simulink library "AEMS_Standard_Library"  (R2016b)
settings: Solver=ode45  StartTime=0.0  StopTime=10.0  RelTol=1e-3
undefined symbols (not defined in the file or in its folder): BkPY, carto, Cbx_extegr, Cbx_lpegrsys, Cbx_portegr, Cnx_bnk_nr_conf, Cnx_cyl_nr_conf, ConfigManagement, configuration_management, Cxx_dcm_io_tmr_end_xxxx, Cxx_dcm_rt_tmr_end, Cxx_DID_xxxx_IO_max, Cxx_DID_xxxx_IO_min, Cxx_egrhsofs, Cxx_vmaniegi, DEM_DEBOUNCE_FREEZE, DEM_DTR_CTL_INVISIBLE, DEM_DTR_CTL_NORMAL, Dem_DtrId2_XXX, Dem_DtrId3_XXX, Dem_DtrId4_XXX, Dem_DtrId5_XXX, Dem_DtrId6_XXX, Dem_DtrId7_XXX, Dem_DtrId8_XXX, Dem_DtrId9_XXX, Dem_DtrId_XXX, Dem_EnableConditionId2_XXX, Dem_EnableConditionId3_XXX, Dem_EnableConditionId4_XXX, Dem_EnableConditionId5_XXX, Dem_EnableConditionId6_XXX, Dem_EnableConditionId7_XXX, Dem_EnableConditionId8_XXX, Dem_EnableConditionId_XXX, Dem_EventId, Dem_EventId2_XXX, Dem_EventId3_XXX, Dem_EventId4_XXX, Dem_EventId5_XXX, Dem_EventId6_XXX, Dem_EventId7_XXX, Dem_EventId8_XXX, Dem_EventId9_XXX, Dem_EventId_Device_Faulttype, Dem_EventId_XXX, DEM_IUMPR_GENERAL_DENOMINATOR, DEM_OPCYC_IGNITION, Dem_RatioId2_XXX, Dem_RatioId3_XXX, Dem_RatioId4_XXX, Dem_RatioId5_XXX, Dem_RatioId6_XXX, Dem_RatioId7_XXX, Dem_RatioId8_XXX, Dem_RatioId_XXX, Dem_StorageConditionId2_XXX, Dem_StorageConditionId3_XXX, Dem_StorageConditionId4_XXX, Dem_StorageConditionId5_XXX ... (+65)
libraries: AEMS_Standard_Library x477, simulink x2
(part 21 of 39)

== system AEMS_Standard_Library/SUB/AEMS_DEM_COUNTER_BASED_DEBOUNCE_6D ==
  note: DemDebounceBehavior
  flag_set : Inport
  conditionfulfilled : Inport  Port=2
  prefailed : Inport  Port=3
  prepassed : Inport  Port=4
  reseteventdebounce : Inport  Port=5
  AEMS_DEM_COUNTER_BASED_DEBOUNCE_CALL1 : Subsystem
  AEMS_DEM_COUNTER_BASED_DEBOUNCE_CALL2 : Subsystem
  AEMS_DEM_COUNTER_BASED_DEBOUNCE_CALL3 : Subsystem
  AEMS_DEM_COUNTER_BASED_DEBOUNCE_CALL4 : Subsystem
  AEMS_DEM_COUNTER_BASED_DEBOUNCE_CALL5 : Subsystem
  AEMS_DEM_COUNTER_BASED_DEBOUNCE_CALL6 : Subsystem
  DemCounterDecrementStepSize : Constant  Value=DemCounterDecrementStepSize
  DemCounterFailedThreshold : Constant  Value=DemCounterFailedThreshold
  DemCounterIncrementStepSize : Constant  Value=DemCounterIncrementStepSize
  DemCounterJumpDown : Constant  Value=DemCounterJumpDown
  DemCounterJumpDownValue : Constant  Value=DemCounterJumpDownValue
  DemCounterJumpUp : Constant  Value=DemCounterJumpUp
  DemCounterJumpUpValue : Constant  Value=DemCounterJumpUpValue
  DemCounterPassedThreshold : Constant  Value=DemCounterPassedThreshold
  DemDebounceBehavior : Constant  Value=[0,0,0,0,0,0]  OutDataTypeStr=uint8
  Demux{,1..13} (14 alike) : Demux  Outputs=6
  Mux : Mux  Inputs=6
  Mux1 : Mux  Inputs=6
  Mux2 : Mux  Inputs=6
  debouncevalue : Outport
  failed : Outport  Port=2
  passed : Outport  Port=3
  wires:
  AEMS_DEM_COUNTER_BASED_DEBOUNCE_CALL6/3(passed) -> Mux/6
  AEMS_DEM_COUNTER_BASED_DEBOUNCE_CALL5/3(passed) -> Mux/5
  AEMS_DEM_COUNTER_BASED_DEBOUNCE_CALL6/2(failed) -> Mux2/6
  AEMS_DEM_COUNTER_BASED_DEBOUNCE_CALL5/2(failed) -> Mux2/5
  AEMS_DEM_COUNTER_BASED_DEBOUNCE_CALL6/1(debouncevalue) -> Mux1/6
  AEMS_DEM_COUNTER_BASED_DEBOUNCE_CALL5/1(debouncevalue) -> Mux1/5
  Demux7/6 -> AEMS_DEM_COUNTER_BASED_DEBOUNCE_CALL6/13(DemCounterJumpDownValue)
  Demux7/5 -> AEMS_DEM_COUNTER_BASED_DEBOUNCE_CALL5/13(DemCounterJumpDownValue)
  Demux6/6 -> AEMS_DEM_COUNTER_BASED_DEBOUNCE_CALL6/12(DemCounterJumpDown)
  Demux6/5 -> AEMS_DEM_COUNTER_BASED_DEBOUNCE_CALL5/12(DemCounterJumpDown)
  Demux5/6 -> AEMS_DEM_COUNTER_BASED_DEBOUNCE_CALL6/11(DemCounterDecrementStepSize)
  Demux5/5 -> AEMS_DEM_COUNTER_BASED_DEBOUNCE_CALL5/11(DemCounterDecrementStepSize)
  Demux10/6 -> AEMS_DEM_COUNTER_BASED_DEBOUNCE_CALL6/10(DemCounterPassedThreshold)
  Demux10/5 -> AEMS_DEM_COUNTER_BASED_DEBOUNCE_CALL5/10(DemCounterPassedThreshold)
  Demux9/6 -> AEMS_DEM_COUNTER_BASED_DEBOUNCE_CALL6/9(DemCounterJumpUpValue)
  Demux9/5 -> AEMS_DEM_COUNTER_BASED_DEBOUNCE_CALL5/9(DemCounterJumpUpValue)
  Demux8/6 -> AEMS_DEM_COUNTER_BASED_DEBOUNCE_CALL6/8(DemCounterJumpUp)
  Demux8/5 -> AEMS_DEM_COUNTER_BASED_DEBOUNCE_CALL5/8(DemCounterJumpUp)
  Demux13/6 -> AEMS_DEM_COUNTER_BASED_DEBOUNCE_CALL6/7(DemCounterIncrementStepSize)
  Demux13/5 -> AEMS_DEM_COUNTER_BASED_DEBOUNCE_CALL5/7(DemCounterIncrementStepSize)
  Demux12/6 -> AEMS_DEM_COUNTER_BASED_DEBOUNCE_CALL6/6(DemCounterFailedThreshold)
  Demux12/5 -> AEMS_DEM_COUNTER_BASED_DEBOUNCE_CALL5/6(DemCounterFailedThreshold)
  Demux11/6 -> AEMS_DEM_COUNTER_BASED_DEBOUNCE_CALL6/5(DemDebounceBehavior)
  Demux11/5 -> AEMS_DEM_COUNTER_BASED_DEBOUNCE_CALL5/5(DemDebounceBehavior)
  Demux4/6 -> AEMS_DEM_COUNTER_BASED_DEBOUNCE_CALL6/4(reseteventdebounce)
  Demux4/5 -> AEMS_DEM_COUNTER_BASED_DEBOUNCE_CALL5/4(reseteventdebounce)
  Demux3/6 -> AEMS_DEM_COUNTER_BASED_DEBOUNCE_CALL6/3(prepassed)
  Demux3/5 -> AEMS_DEM_COUNTER_BASED_DEBOUNCE_CALL5/3(prepassed)
  Demux2/6 -> AEMS_DEM_COUNTER_BASED_DEBOUNCE_CALL6/2(prefailed)
  Demux2/5 -> AEMS_DEM_COUNTER_BASED_DEBOUNCE_CALL5/2(prefailed)
  Demux1/6 -> AEMS_DEM_COUNTER_BASED_DEBOUNCE_CALL6/1(conditionfulfilled)
  Demux1/5 -> AEMS_DEM_COUNTER_BASED_DEBOUNCE_CALL5/1(conditionfulfilled)
  Demux/6 -> AEMS_DEM_COUNTER_BASED_DEBOUNCE_CALL6/Enable
  Demux/5 -> AEMS_DEM_COUNTER_BASED_DEBOUNCE_CALL5/Enable
  AEMS_DEM_COUNTER_BASED_DEBOUNCE_CALL4/3(passed) -> Mux/4
  AEMS_DEM_COUNTER_BASED_DEBOUNCE_CALL4/2(failed) -> Mux2/4
  AEMS_DEM_COUNTER_BASED_DEBOUNCE_CALL4/1(debouncevalue) -> Mux1/4
  Demux7/4 -> AEMS_DEM_COUNTER_BASED_DEBOUNCE_CALL4/13(DemCounterJumpDownValue)
  Demux6/4 -> AEMS_DEM_COUNTER_BASED_DEBOUNCE_CALL4/12(DemCounterJumpDown)
  Demux5/4 -> AEMS_DEM_COUNTER_BASED_DEBOUNCE_CALL4/11(DemCounterDecrementStepSize)
  Demux10/4 -> AEMS_DEM_COUNTER_BASED_DEBOUNCE_CALL4/10(DemCounterPassedThreshold)
  Demux9/4 -> AEMS_DEM_COUNTER_BASED_DEBOUNCE_CALL4/9(DemCounterJumpUpValue)
  Demux8/4 -> AEMS_DEM_COUNTER_BASED_DEBOUNCE_CALL4/8(DemCounterJumpUp)
  Demux13/4 -> AEMS_DEM_COUNTER_BASED_DEBOUNCE_CALL4/7(DemCounterIncrementStepSize)
  Demux12/4 -> AEMS_DEM_COUNTER_BASED_DEBOUNCE_CALL4/6(DemCounterFailedThreshold)
  Demux11/4 -> AEMS_DEM_COUNTER_BASED_DEBOUNCE_CALL4/5(DemDebounceBehavior)
  Demux4/4 -> AEMS_DEM_COUNTER_BASED_DEBOUNCE_CALL4/4(reseteventdebounce)
  Demux3/4 -> AEMS_DEM_COUNTER_BASED_DEBOUNCE_CALL4/3(prepassed)
  Demux2/4 -> AEMS_DEM_COUNTER_BASED_DEBOUNCE_CALL4/2(prefailed)
  Demux1/4 -> AEMS_DEM_COUNTER_BASED_DEBOUNCE_CALL4/1(conditionfulfilled)
  Demux/4 -> AEMS_DEM_COUNTER_BASED_DEBOUNCE_CALL4/Enable
  flag_set/1 -> Demux/1
  conditionfulfilled/1 -> Demux1/1  "conditionfulfilled"
  prefailed/1 -> Demux2/1  "prefailed"
  prepassed/1 -> Demux3/1  "prepassed"
  reseteventdebounce/1 -> Demux4/1  "reseteventdebounce"
  DemCounterDecrementStepSize/1 -> Demux5/1  "decrementstepsize_for_prepassed"
  DemCounterJumpDown/1 -> Demux6/1  "jumpdown_activation_with_prepassed"
  DemCounterJumpDownValue/1 -> Demux7/1  "jumpupvalue_with_prefailed"
  DemCounterJumpUp/1 -> Demux8/1  "jumpup_activation_with_prefailed"
  DemCounterJumpUpValue/1 -> Demux9/1  "jumpupvalue_with_prefailed"
  DemCounterPassedThreshold/1 -> Demux10/1  "passedthreshold"
  DemDebounceBehavior/1 -> Demux11/1  "behavior"
  DemCounterFailedThreshold/1 -> Demux12/1  "failedthreshold"
  DemCounterIncrementStepSize/1 -> Demux13/1  "incrementstepsize_for_prefailed"
  Demux7/2 -> AEMS_DEM_COUNTER_BASED_DEBOUNCE_CALL2/13(DemCounterJumpDownValue)
  Demux6/2 -> AEMS_DEM_COUNTER_BASED_DEBOUNCE_CALL2/12(DemCounterJumpDown)
  Demux5/2 -> AEMS_DEM_COUNTER_BASED_DEBOUNCE_CALL2/11(DemCounterDecrementStepSize)
  Demux10/2 -> AEMS_DEM_COUNTER_BASED_DEBOUNCE_CALL2/10(DemCounterPassedThreshold)
  Demux9/2 -> AEMS_DEM_COUNTER_BASED_DEBOUNCE_CALL2/9(DemCounterJumpUpValue)
  Demux8/2 -> AEMS_DEM_COUNTER_BASED_DEBOUNCE_CALL2/8(DemCounterJumpUp)
  Demux13/2 -> AEMS_DEM_COUNTER_BASED_DEBOUNCE_CALL2/7(DemCounterIncrementStepSize)
  Demux12/2 -> AEMS_DEM_COUNTER_BASED_DEBOUNCE_CALL2/6(DemCounterFailedThreshold)
  Demux11/2 -> AEMS_DEM_COUNTER_BASED_DEBOUNCE_CALL2/5(DemDebounceBehavior)
  Demux4/2 -> AEMS_DEM_COUNTER_BASED_DEBOUNCE_CALL2/4(reseteventdebounce)
  Demux3/2 -> AEMS_DEM_COUNTER_BASED_DEBOUNCE_CALL2/3(prepassed)
  Demux2/2 -> AEMS_DEM_COUNTER_BASED_DEBOUNCE_CALL2/2(prefailed)
  Demux1/2 -> AEMS_DEM_COUNTER_BASED_DEBOUNCE_CALL2/1(conditionfulfilled)
  Demux/2 -> AEMS_DEM_COUNTER_BASED_DEBOUNCE_CALL2/Enable
  Demux/1 -> AEMS_DEM_COUNTER_BASED_DEBOUNCE_CALL1/Enable
  Demux1/1 -> AEMS_DEM_COUNTER_BASED_DEBOUNCE_CALL1/1(conditionfulfilled)
  Demux2/1 -> AEMS_DEM_COUNTER_BASED_DEBOUNCE_CALL1/2(prefailed)
  Demux3/1 -> AEMS_DEM_COUNTER_BASED_DEBOUNCE_CALL1/3(prepassed)
  Demux4/1 -> AEMS_DEM_COUNTER_BASED_DEBOUNCE_CALL1/4(reseteventdebounce)
  Demux11/1 -> AEMS_DEM_COUNTER_BASED_DEBOUNCE_CALL1/5(DemDebounceBehavior)
  Demux12/1 -> AEMS_DEM_COUNTER_BASED_DEBOUNCE_CALL1/6(DemCounterFailedThreshold)
  Demux13/1 -> AEMS_DEM_COUNTER_BASED_DEBOUNCE_CALL1/7(DemCounterIncrementStepSize)
  Demux8/1 -> AEMS_DEM_COUNTER_BASED_DEBOUNCE_CALL1/8(DemCounterJumpUp)
  Demux9/1 -> AEMS_DEM_COUNTER_BASED_DEBOUNCE_CALL1/9(DemCounterJumpUpValue)
  Demux10/1 -> AEMS_DEM_COUNTER_BASED_DEBOUNCE_CALL1/10(DemCounterPassedThreshold)
  Demux5/1 -> AEMS_DEM_COUNTER_BASED_DEBOUNCE_CALL1/11(DemCounterDecrementStepSize)
  Demux6/1 -> AEMS_DEM_COUNTER_BASED_DEBOUNCE_CALL1/12(DemCounterJumpDown)
  Demux7/1 -> AEMS_DEM_COUNTER_BASED_DEBOUNCE_CALL1/13(DemCounterJumpDownValue)
  Mux/1 -> passed/1
  Mux1/1 -> debouncevalue/1
  Mux2/1 -> failed/1
  AEMS_DEM_COUNTER_BASED_DEBOUNCE_CALL1/1(debouncevalue) -> Mux1/1
  AEMS_DEM_COUNTER_BASED_DEBOUNCE_CALL1/2(failed) -> Mux2/1
  AEMS_DEM_COUNTER_BASED_DEBOUNCE_CALL1/3(passed) -> Mux/1
  AEMS_DEM_COUNTER_BASED_DEBOUNCE_CALL2/1(debouncevalue) -> Mux1/2
  AEMS_DEM_COUNTER_BASED_DEBOUNCE_CALL2/2(failed) -> Mux2/2
  AEMS_DEM_COUNTER_BASED_DEBOUNCE_CALL2/3(passed) -> Mux/2
  Demux/3 -> AEMS_DEM_COUNTER_BASED_DEBOUNCE_CALL3/Enable
  Demux1/3 -> AEMS_DEM_COUNTER_BASED_DEBOUNCE_CALL3/1(conditionfulfilled)
  Demux2/3 -> AEMS_DEM_COUNTER_BASED_DEBOUNCE_CALL3/2(prefailed)
  Demux3/3 -> AEMS_DEM_COUNTER_BASED_DEBOUNCE_CALL3/3(prepassed)
  Demux4/3 -> AEMS_DEM_COUNTER_BASED_DEBOUNCE_CALL3/4(reseteventdebounce)
  Demux11/3 -> AEMS_DEM_COUNTER_BASED_DEBOUNCE_CALL3/5(DemDebounceBehavior)
  Demux12/3 -> AEMS_DEM_COUNTER_BASED_DEBOUNCE_CALL3/6(DemCounterFailedThreshold)
  Demux13/3 -> AEMS_DEM_COUNTER_BASED_DEBOUNCE_CALL3/7(DemCounterIncrementStepSize)
  Demux8/3 -> AEMS_DEM_COUNTER_BASED_DEBOUNCE_CALL3/8(DemCounterJumpUp)
  Demux9/3 -> AEMS_DEM_COUNTER_BASED_DEBOUNCE_CALL3/9(DemCounterJumpUpValue)
  Demux10/3 -> AEMS_DEM_COUNTER_BASED_DEBOUNCE_CALL3/10(DemCounterPassedThreshold)
  Demux5/3 -> AEMS_DEM_COUNTER_BASED_DEBOUNCE_CALL3/11(DemCounterDecrementStepSize)
  Demux6/3 -> AEMS_DEM_COUNTER_BASED_DEBOUNCE_CALL3/12(DemCounterJumpDown)
  Demux7/3 -> AEMS_DEM_COUNTER_BASED_DEBOUNCE_CALL3/13(DemCounterJumpDownValue)
  AEMS_DEM_COUNTER_BASED_DEBOUNCE_CALL3/1(debouncevalue) -> Mux1/3
  AEMS_DEM_COUNTER_BASED_DEBOUNCE_CALL3/2(failed) -> Mux2/3
  AEMS_DEM_COUNTER_BASED_DEBOUNCE_CALL3/3(passed) -> Mux/3

== system AEMS_Standard_Library/SUB/AEMS_DEM_COUNTER_BASED_DEBOUNCE_8D ==
  note: DemDebounceBehavior
  flag_set : Inport
  conditionfulfilled : Inport  Port=2
  prefailed : Inport  Port=3
  prepassed : Inport  Port=4
  reseteventdebounce : Inport  Port=5
  AEMS_DEM_COUNTER_BASED_DEBOUNCE_CALL1 : Subsystem
  AEMS_DEM_COUNTER_BASED_DEBOUNCE_CALL2 : Subsystem
  AEMS_DEM_COUNTER_BASED_DEBOUNCE_CALL3 : Subsystem
  AEMS_DEM_COUNTER_BASED_DEBOUNCE_CALL4 : Subsystem
  AEMS_DEM_COUNTER_BASED_DEBOUNCE_CALL5 : Subsystem
  AEMS_DEM_COUNTER_BASED_DEBOUNCE_CALL6 : Subsystem
  AEMS_DEM_COUNTER_BASED_DEBOUNCE_CALL7 : Subsystem
  AEMS_DEM_COUNTER_BASED_DEBOUNCE_CALL8 : Subsystem
  DemCounterDecrementStepSize : Constant  Value=DemCounterDecrementStepSize
  DemCounterFailedThreshold : Constant  Value=DemCounterFailedThreshold
  DemCounterIncrementStepSize : Constant  Value=DemCounterIncrementStepSize
  DemCounterJumpDown : Constant  Value=DemCounterJumpDown
  DemCounterJumpDownValue : Constant  Value=DemCounterJumpDownValue
  DemCounterJumpUp : Constant  Value=DemCounterJumpUp
  DemCounterJumpUpValue : Constant  Value=DemCounterJumpUpValue
  DemCounterPassedThreshold : Constant  Value=DemCounterPassedThreshold
  DemDebounceBehavior : Constant  Value=[0,0,0,0,0,0,0,0]  OutDataTypeStr=uint8
  Demux{,1..13} (14 alike) : Demux  Outputs=8
  Mux : Mux  Inputs=8
  Mux1 : Mux  Inputs=8
  Mux2 : Mux  Inputs=8
  debouncevalue : Outport
  failed : Outport  Port=2
  passed : Outport  Port=3
  wires:
  AEMS_DEM_COUNTER_BASED_DEBOUNCE_CALL8/3(passed) -> Mux/8
  AEMS_DEM_COUNTER_BASED_DEBOUNCE_CALL7/3(passed) -> Mux/7
  AEMS_DEM_COUNTER_BASED_DEBOUNCE_CALL8/2(failed) -> Mux2/8
  AEMS_DEM_COUNTER_BASED_DEBOUNCE_CALL7/2(failed) -> Mux2/7
  AEMS_DEM_COUNTER_BASED_DEBOUNCE_CALL8/1(debouncevalue) -> Mux1/8
  AEMS_DEM_COUNTER_BASED_DEBOUNCE_CALL7/1(debouncevalue) -> Mux1/7
  Demux7/8 -> AEMS_DEM_COUNTER_BASED_DEBOUNCE_CALL8/13(DemCounterJumpDownValue)
  Demux7/7 -> AEMS_DEM_COUNTER_BASED_DEBOUNCE_CALL7/13(DemCounterJumpDownValue)
  Demux6/8 -> AEMS_DEM_COUNTER_BASED_DEBOUNCE_CALL8/12(DemCounterJumpDown)
  Demux6/7 -> AEMS_DEM_COUNTER_BASED_DEBOUNCE_CALL7/12(DemCounterJumpDown)
  Demux5/8 -> AEMS_DEM_COUNTER_BASED_DEBOUNCE_CALL8/11(DemCounterDecrementStepSize)
  Demux5/7 -> AEMS_DEM_COUNTER_BASED_DEBOUNCE_CALL7/11(DemCounterDecrementStepSize)
  Demux10/8 -> AEMS_DEM_COUNTER_BASED_DEBOUNCE_CALL8/10(DemCounterPassedThreshold)
  Demux10/7 -> AEMS_DEM_COUNTER_BASED_DEBOUNCE_CALL7/10(DemCounterPassedThreshold)
  Demux9/8 -> AEMS_DEM_COUNTER_BASED_DEBOUNCE_CALL8/9(DemCounterJumpUpValue)
  Demux9/7 -> AEMS_DEM_COUNTER_BASED_DEBOUNCE_CALL7/9(DemCounterJumpUpValue)
  Demux8/8 -> AEMS_DEM_COUNTER_BASED_DEBOUNCE_CALL8/8(DemCounterJumpUp)
  Demux8/7 -> AEMS_DEM_COUNTER_BASED_DEBOUNCE_CALL7/8(DemCounterJumpUp)
  Demux13/8 -> AEMS_DEM_COUNTER_BASED_DEBOUNCE_CALL8/7(DemCounterIncrementStepSize)
  Demux13/7 -> AEMS_DEM_COUNTER_BASED_DEBOUNCE_CALL7/7(DemCounterIncrementStepSize)
  Demux12/8 -> AEMS_DEM_COUNTER_BASED_DEBOUNCE_CALL8/6(DemCounterFailedThreshold)
  Demux12/7 -> AEMS_DEM_COUNTER_BASED_DEBOUNCE_CALL7/6(DemCounterFailedThreshold)
  Demux11/8 -> AEMS_DEM_COUNTER_BASED_DEBOUNCE_CALL8/5(DemDebounceBehavior)
  Demux11/7 -> AEMS_DEM_COUNTER_BASED_DEBOUNCE_CALL7/5(DemDebounceBehavior)
  Demux4/8 -> AEMS_DEM_COUNTER_BASED_DEBOUNCE_CALL8/4(reseteventdebounce)
  Demux4/7 -> AEMS_DEM_COUNTER_BASED_DEBOUNCE_CALL7/4(reseteventdebounce)
  Demux3/8 -> AEMS_DEM_COUNTER_BASED_DEBOUNCE_CALL8/3(prepassed)
  Demux3/7 -> AEMS_DEM_COUNTER_BASED_DEBOUNCE_CALL7/3(prepassed)
  Demux2/8 -> AEMS_DEM_COUNTER_BASED_DEBOUNCE_CALL8/2(prefailed)
  Demux2/7 -> AEMS_DEM_COUNTER_BASED_DEBOUNCE_CALL7/2(prefailed)
  Demux1/8 -> AEMS_DEM_COUNTER_BASED_DEBOUNCE_CALL8/1(conditionfulfilled)
  Demux1/7 -> AEMS_DEM_COUNTER_BASED_DEBOUNCE_CALL7/1(conditionfulfilled)
  Demux/8 -> AEMS_DEM_COUNTER_BASED_DEBOUNCE_CALL8/Enable
  Demux/7 -> AEMS_DEM_COUNTER_BASED_DEBOUNCE_CALL7/Enable
  AEMS_DEM_COUNTER_BASED_DEBOUNCE_CALL6/3(passed) -> Mux/6
  AEMS_DEM_COUNTER_BASED_DEBOUNCE_CALL5/3(passed) -> Mux/5
  AEMS_DEM_COUNTER_BASED_DEBOUNCE_CALL6/2(failed) -> Mux2/6
  AEMS_DEM_COUNTER_BASED_DEBOUNCE_CALL5/2(failed) -> Mux2/5
  AEMS_DEM_COUNTER_BASED_DEBOUNCE_CALL6/1(debouncevalue) -> Mux1/6
  AEMS_DEM_COUNTER_BASED_DEBOUNCE_CALL5/1(debouncevalue) -> Mux1/5
  Demux7/6 -> AEMS_DEM_COUNTER_BASED_DEBOUNCE_CALL6/13(DemCounterJumpDownValue)
  Demux7/5 -> AEMS_DEM_COUNTER_BASED_DEBOUNCE_CALL5/13(DemCounterJumpDownValue)
  Demux6/6 -> AEMS_DEM_COUNTER_BASED_DEBOUNCE_CALL6/12(DemCounterJumpDown)
  Demux6/5 -> AEMS_DEM_COUNTER_BASED_DEBOUNCE_CALL5/12(DemCounterJumpDown)
  Demux5/6 -> AEMS_DEM_COUNTER_BASED_DEBOUNCE_CALL6/11(DemCounterDecrementStepSize)
  Demux5/5 -> AEMS_DEM_COUNTER_BASED_DEBOUNCE_CALL5/11(DemCounterDecrementStepSize)
  Demux10/6 -> AEMS_DEM_COUNTER_BASED_DEBOUNCE_CALL6/10(DemCounterPassedThreshold)
  Demux10/5 -> AEMS_DEM_COUNTER_BASED_DEBOUNCE_CALL5/10(DemCounterPassedThreshold)
  Demux9/6 -> AEMS_DEM_COUNTER_BASED_DEBOUNCE_CALL6/9(DemCounterJumpUpValue)
  Demux9/5 -> AEMS_DEM_COUNTER_BASED_DEBOUNCE_CALL5/9(DemCounterJumpUpValue)
  Demux8/6 -> AEMS_DEM_COUNTER_BASED_DEBOUNCE_CALL6/8(DemCounterJumpUp)
  Demux8/5 -> AEMS_DEM_COUNTER_BASED_DEBOUNCE_CALL5/8(DemCounterJumpUp)
  Demux13/6 -> AEMS_DEM_COUNTER_BASED_DEBOUNCE_CALL6/7(DemCounterIncrementStepSize)
  Demux13/5 -> AEMS_DEM_COUNTER_BASED_DEBOUNCE_CALL5/7(DemCounterIncrementStepSize)
  Demux12/6 -> AEMS_DEM_COUNTER_BASED_DEBOUNCE_CALL6/6(DemCounterFailedThreshold)
  Demux12/5 -> AEMS_DEM_COUNTER_BASED_DEBOUNCE_CALL5/6(DemCounterFailedThreshold)
  Demux11/6 -> AEMS_DEM_COUNTER_BASED_DEBOUNCE_CALL6/5(DemDebounceBehavior)
  Demux11/5 -> AEMS_DEM_COUNTER_BASED_DEBOUNCE_CALL5/5(DemDebounceBehavior)
  Demux4/6 -> AEMS_DEM_COUNTER_BASED_DEBOUNCE_CALL6/4(reseteventdebounce)
  Demux4/5 -> AEMS_DEM_COUNTER_BASED_DEBOUNCE_CALL5/4(reseteventdebounce)
  Demux3/6 -> AEMS_DEM_COUNTER_BASED_DEBOUNCE_CALL6/3(prepassed)
  Demux3/5 -> AEMS_DEM_COUNTER_BASED_DEBOUNCE_CALL5/3(prepassed)
  Demux2/6 -> AEMS_DEM_COUNTER_BASED_DEBOUNCE_CALL6/2(prefailed)
  Demux2/5 -> AEMS_DEM_COUNTER_BASED_DEBOUNCE_CALL5/2(prefailed)
  Demux1/6 -> AEMS_DEM_COUNTER_BASED_DEBOUNCE_CALL6/1(conditionfulfilled)
  Demux1/5 -> AEMS_DEM_COUNTER_BASED_DEBOUNCE_CALL5/1(conditionfulfilled)
  Demux/6 -> AEMS_DEM_COUNTER_BASED_DEBOUNCE_CALL6/Enable
  Demux/5 -> AEMS_DEM_COUNTER_BASED_DEBOUNCE_CALL5/Enable
  AEMS_DEM_COUNTER_BASED_DEBOUNCE_CALL4/3(passed) -> Mux/4
  AEMS_DEM_COUNTER_BASED_DEBOUNCE_CALL4/2(failed) -> Mux2/4
  AEMS_DEM_COUNTER_BASED_DEBOUNCE_CALL4/1(debouncevalue) -> Mux1/4
  Demux7/4 -> AEMS_DEM_COUNTER_BASED_DEBOUNCE_CALL4/13(DemCounterJumpDownValue)
  Demux6/4 -> AEMS_DEM_COUNTER_BASED_DEBOUNCE_CALL4/12(DemCounterJumpDown)
  Demux5/4 -> AEMS_DEM_COUNTER_BASED_DEBOUNCE_CALL4/11(DemCounterDecrementStepSize)
  Demux10/4 -> AEMS_DEM_COUNTER_BASED_DEBOUNCE_CALL4/10(DemCounterPassedThreshold)
  Demux9/4 -> AEMS_DEM_COUNTER_BASED_DEBOUNCE_CALL4/9(DemCounterJumpUpValue)
  Demux8/4 -> AEMS_DEM_COUNTER_BASED_DEBOUNCE_CALL4/8(DemCounterJumpUp)
  Demux13/4 -> AEMS_DEM_COUNTER_BASED_DEBOUNCE_CALL4/7(DemCounterIncrementStepSize)
  Demux12/4 -> AEMS_DEM_COUNTER_BASED_DEBOUNCE_CALL4/6(DemCounterFailedThreshold)
  Demux11/4 -> AEMS_DEM_COUNTER_BASED_DEBOUNCE_CALL4/5(DemDebounceBehavior)
  Demux4/4 -> AEMS_DEM_COUNTER_BASED_DEBOUNCE_CALL4/4(reseteventdebounce)
  Demux3/4 -> AEMS_DEM_COUNTER_BASED_DEBOUNCE_CALL4/3(prepassed)
  Demux2/4 -> AEMS_DEM_COUNTER_BASED_DEBOUNCE_CALL4/2(prefailed)
  Demux1/4 -> AEMS_DEM_COUNTER_BASED_DEBOUNCE_CALL4/1(conditionfulfilled)
  Demux/4 -> AEMS_DEM_COUNTER_BASED_DEBOUNCE_CALL4/Enable
  flag_set/1 -> Demux/1
  conditionfulfilled/1 -> Demux1/1  "conditionfulfilled"
  prefailed/1 -> Demux2/1  "prefailed"
  prepassed/1 -> Demux3/1  "prepassed"
  reseteventdebounce/1 -> Demux4/1  "reseteventdebounce"
  DemCounterDecrementStepSize/1 -> Demux5/1  "decrementstepsize_for_prepassed"
  DemCounterJumpDown/1 -> Demux6/1  "jumpdown_activation_with_prepassed"
  DemCounterJumpDownValue/1 -> Demux7/1  "jumpupvalue_with_prefailed"
  DemCounterJumpUp/1 -> Demux8/1  "jumpup_activation_with_prefailed"
  DemCounterJumpUpValue/1 -> Demux9/1  "jumpupvalue_with_prefailed"
  DemCounterPassedThreshold/1 -> Demux10/1  "passedthreshold"
  DemDebounceBehavior/1 -> Demux11/1  "behavior"
  DemCounterFailedThreshold/1 -> Demux12/1  "failedthreshold"
  DemCounterIncrementStepSize/1 -> Demux13/1  "incrementstepsize_for_prefailed"
  Demux7/2 -> AEMS_DEM_COUNTER_BASED_DEBOUNCE_CALL2/13(DemCounterJumpDownValue)
  Demux6/2 -> AEMS_DEM_COUNTER_BASED_DEBOUNCE_CALL2/12(DemCounterJumpDown)
  Demux5/2 -> AEMS_DEM_COUNTER_BASED_DEBOUNCE_CALL2/11(DemCounterDecrementStepSize)
  Demux10/2 -> AEMS_DEM_COUNTER_BASED_DEBOUNCE_CALL2/10(DemCounterPassedThreshold)
  Demux9/2 -> AEMS_DEM_COUNTER_BASED_DEBOUNCE_CALL2/9(DemCounterJumpUpValue)
  Demux8/2 -> AEMS_DEM_COUNTER_BASED_DEBOUNCE_CALL2/8(DemCounterJumpUp)
  Demux13/2 -> AEMS_DEM_COUNTER_BASED_DEBOUNCE_CALL2/7(DemCounterIncrementStepSize)
  Demux12/2 -> AEMS_DEM_COUNTER_BASED_DEBOUNCE_CALL2/6(DemCounterFailedThreshold)
  Demux11/2 -> AEMS_DEM_COUNTER_BASED_DEBOUNCE_CALL2/5(DemDebounceBehavior)
  Demux4/2 -> AEMS_DEM_COUNTER_BASED_DEBOUNCE_CALL2/4(reseteventdebounce)
  Demux3/2 -> AEMS_DEM_COUNTER_BASED_DEBOUNCE_CALL2/3(prepassed)
  Demux2/2 -> AEMS_DEM_COUNTER_BASED_DEBOUNCE_CALL2/2(prefailed)
  Demux1/2 -> AEMS_DEM_COUNTER_BASED_DEBOUNCE_CALL2/1(conditionfulfilled)
  Demux/2 -> AEMS_DEM_COUNTER_BASED_DEBOUNCE_CALL2/Enable
  Demux/1 -> AEMS_DEM_COUNTER_BASED_DEBOUNCE_CALL1/Enable
  Demux1/1 -> AEMS_DEM_COUNTER_BASED_DEBOUNCE_CALL1/1(conditionfulfilled)
  Demux2/1 -> AEMS_DEM_COUNTER_BASED_DEBOUNCE_CALL1/2(prefailed)
  Demux3/1 -> AEMS_DEM_COUNTER_BASED_DEBOUNCE_CALL1/3(prepassed)
  Demux4/1 -> AEMS_DEM_COUNTER_BASED_DEBOUNCE_CALL1/4(reseteventdebounce)
  Demux11/1 -> AEMS_DEM_COUNTER_BASED_DEBOUNCE_CALL1/5(DemDebounceBehavior)
  Demux12/1 -> AEMS_DEM_COUNTER_BASED_DEBOUNCE_CALL1/6(DemCounterFailedThreshold)
  Demux13/1 -> AEMS_DEM_COUNTER_BASED_DEBOUNCE_CALL1/7(DemCounterIncrementStepSize)
  Demux8/1 -> AEMS_DEM_COUNTER_BASED_DEBOUNCE_CALL1/8(DemCounterJumpUp)
  Demux9/1 -> AEMS_DEM_COUNTER_BASED_DEBOUNCE_CALL1/9(DemCounterJumpUpValue)
  Demux10/1 -> AEMS_DEM_COUNTER_BASED_DEBOUNCE_CALL1/10(DemCounterPassedThreshold)
  Demux5/1 -> AEMS_DEM_COUNTER_BASED_DEBOUNCE_CALL1/11(DemCounterDecrementStepSize)
  Demux6/1 -> AEMS_DEM_COUNTER_BASED_DEBOUNCE_CALL1/12(DemCounterJumpDown)
  Demux7/1 -> AEMS_DEM_COUNTER_BASED_DEBOUNCE_CALL1/13(DemCounterJumpDownValue)
  Mux/1 -> passed/1
  Mux1/1 -> debouncevalue/1
  Mux2/1 -> failed/1
  AEMS_DEM_COUNTER_BASED_DEBOUNCE_CALL1/1(debouncevalue) -> Mux1/1
  AEMS_DEM_COUNTER_BASED_DEBOUNCE_CALL1/2(failed) -> Mux2/1
  AEMS_DEM_COUNTER_BASED_DEBOUNCE_CALL1/3(passed) -> Mux/1
  AEMS_DEM_COUNTER_BASED_DEBOUNCE_CALL2/1(debouncevalue) -> Mux1/2
  AEMS_DEM_COUNTER_BASED_DEBOUNCE_CALL2/2(failed) -> Mux2/2
  AEMS_DEM_COUNTER_BASED_DEBOUNCE_CALL2/3(passed) -> Mux/2
  Demux/3 -> AEMS_DEM_COUNTER_BASED_DEBOUNCE_CALL3/Enable
  Demux1/3 -> AEMS_DEM_COUNTER_BASED_DEBOUNCE_CALL3/1(conditionfulfilled)
  Demux2/3 -> AEMS_DEM_COUNTER_BASED_DEBOUNCE_CALL3/2(prefailed)
  Demux3/3 -> AEMS_DEM_COUNTER_BASED_DEBOUNCE_CALL3/3(prepassed)
  Demux4/3 -> AEMS_DEM_COUNTER_BASED_DEBOUNCE_CALL3/4(reseteventdebounce)
  Demux11/3 -> AEMS_DEM_COUNTER_BASED_DEBOUNCE_CALL3/5(DemDebounceBehavior)
  Demux12/3 -> AEMS_DEM_COUNTER_BASED_DEBOUNCE_CALL3/6(DemCounterFailedThreshold)
  Demux13/3 -> AEMS_DEM_COUNTER_BASED_DEBOUNCE_CALL3/7(DemCounterIncrementStepSize)
  Demux8/3 -> AEMS_DEM_COUNTER_BASED_DEBOUNCE_CALL3/8(DemCounterJumpUp)
  Demux9/3 -> AEMS_DEM_COUNTER_BASED_DEBOUNCE_CALL3/9(DemCounterJumpUpValue)
  Demux10/3 -> AEMS_DEM_COUNTER_BASED_DEBOUNCE_CALL3/10(DemCounterPassedThreshold)
  Demux5/3 -> AEMS_DEM_COUNTER_BASED_DEBOUNCE_CALL3/11(DemCounterDecrementStepSize)
  Demux6/3 -> AEMS_DEM_COUNTER_BASED_DEBOUNCE_CALL3/12(DemCounterJumpDown)
  Demux7/3 -> AEMS_DEM_COUNTER_BASED_DEBOUNCE_CALL3/13(DemCounterJumpDownValue)
  AEMS_DEM_COUNTER_BASED_DEBOUNCE_CALL3/1(debouncevalue) -> Mux1/3
  AEMS_DEM_COUNTER_BASED_DEBOUNCE_CALL3/2(failed) -> Mux2/3
  AEMS_DEM_COUNTER_BASED_DEBOUNCE_CALL3/3(passed) -> Mux/3

== system AEMS_Standard_Library/SUB/AEMS_DEM_COUNTER_BASED_DEBOUNCE_THRSHOLD_DYN_1D ==
  note: DemDebounceBehavior
  flag_set : Inport
  conditionfulfilled : Inport  Port=2
  prefailed : Inport  Port=3
  prepassed : Inport  Port=4
  failedthreshold : Inport  Port=5
  passedthreshold : Inport  Port=6
  reseteventdebounce : Inport  Port=7
  AEMS_DEM_COUNTER_BASED_DEBOUNCE_THRSHOLD_DYN_CALL : Subsystem
  DemCounterDecrementStepSize : Constant  Value=DemCounterDecrementStepSize
  DemCounterIncrementStepSize : Constant  Value=DemCounterIncrementStepSize
  DemCounterJumpDown : Constant  Value=DemCounterJumpDown
  DemCounterJumpDownValue : Constant  Value=DemCounterJumpDownValue
  DemCounterJumpUp : Constant  Value=DemCounterJumpUp
  DemCounterJumpUpValue : Constant  Value=DemCounterJumpUpValue
  DemDebounceBehavior : Constant  Value=0  OutDataTypeStr=uint8
  debouncevalue : Outport
  failed : Outport  Port=2
  passed : Outport  Port=3
  wires:
  conditionfulfilled/1 -> AEMS_DEM_COUNTER_BASED_DEBOUNCE_THRSHOLD_DYN_CALL/1(conditionfulfilled)  "conditionfulfilled"
  prefailed/1 -> AEMS_DEM_COUNTER_BASED_DEBOUNCE_THRSHOLD_DYN_CALL/2(prefailed)  "prefailed"
  prepassed/1 -> AEMS_DEM_COUNTER_BASED_DEBOUNCE_THRSHOLD_DYN_CALL/3(prepassed)  "prepassed"
  AEMS_DEM_COUNTER_BASED_DEBOUNCE_THRSHOLD_DYN_CALL/1(debouncevalue) -> debouncevalue/1
  AEMS_DEM_COUNTER_BASED_DEBOUNCE_THRSHOLD_DYN_CALL/2(failed) -> failed/1
  AEMS_DEM_COUNTER_BASED_DEBOUNCE_THRSHOLD_DYN_CALL/3(passed) -> passed/1
  flag_set/1 -> AEMS_DEM_COUNTER_BASED_DEBOUNCE_THRSHOLD_DYN_CALL/Enable
  reseteventdebounce/1 -> AEMS_DEM_COUNTER_BASED_DEBOUNCE_THRSHOLD_DYN_CALL/13(reseteventdebounce)  "reseteventdebounce"
  DemCounterJumpDownValue/1 -> AEMS_DEM_COUNTER_BASED_DEBOUNCE_THRSHOLD_DYN_CALL/12(DemCounterJumpDownValue)  "jumpupvalue_with_prefailed"
  DemCounterJumpDown/1 -> AEMS_DEM_COUNTER_BASED_DEBOUNCE_THRSHOLD_DYN_CALL/11(DemCounterJumpDown)  "jumpdown_activation_with_prepassed"
  DemCounterDecrementStepSize/1 -> AEMS_DEM_COUNTER_BASED_DEBOUNCE_THRSHOLD_DYN_CALL/10(DemCounterDecrementStepSize)  "decrementstepsize_for_prepassed"
  passedthreshold/1 -> AEMS_DEM_COUNTER_BASED_DEBOUNCE_THRSHOLD_DYN_CALL/9(passedthreshold)  "passedthreshold"
  DemCounterJumpUpValue/1 -> AEMS_DEM_COUNTER_BASED_DEBOUNCE_THRSHOLD_DYN_CALL/8(DemCounterJumpUpValue)  "jumpupvalue_with_prefailed"
  DemCounterJumpUp/1 -> AEMS_DEM_COUNTER_BASED_DEBOUNCE_THRSHOLD_DYN_CALL/7(DemCounterJumpUp)  "jumpup_activation_with_prefailed"
  DemCounterIncrementStepSize/1 -> AEMS_DEM_COUNTER_BASED_DEBOUNCE_THRSHOLD_DYN_CALL/6(DemCounterIncrementStepSize)  "incrementstepsize_for_prefailed"
  failedthreshold/1 -> AEMS_DEM_COUNTER_BASED_DEBOUNCE_THRSHOLD_DYN_CALL/5(failedthreshold)  "failedthreshold"
  DemDebounceBehavior/1 -> AEMS_DEM_COUNTER_BASED_DEBOUNCE_THRSHOLD_DYN_CALL/4(DemDebounceBehavior)  "behavior"

== system AEMS_Standard_Library/SUB/AEMS_DEM_COUNTER_BASED_DEBOUNCE_THRSHOLD_DYN_2D ==
  note: DemDebounceBehavior
  flag_set : Inport
  conditionfulfilled : Inport  Port=2
  prefailed : Inport  Port=3
  prepassed : Inport  Port=4
  failedthreshold : Inport  Port=5
  passedthreshold : Inport  Port=6
  reseteventdebounce : Inport  Port=7
  AEMS_DEM_COUNTER_BASED_DEBOUNCE_THRSHOLD_DYN_CALL1 : Subsystem
  AEMS_DEM_COUNTER_BASED_DEBOUNCE_THRSHOLD_DYN_CALL2 : Subsystem
  DemCounterDecrementStepSize : Constant  Value=DemCounterDecrementStepSize
  DemCounterIncrementStepSize : Constant  Value=DemCounterIncrementStepSize
  DemCounterJumpDown : Constant  Value=DemCounterJumpDown
  DemCounterJumpDownValue : Constant  Value=DemCounterJumpDownValue
  DemCounterJumpUp : Constant  Value=DemCounterJumpUp
  DemCounterJumpUpValue : Constant  Value=DemCounterJumpUpValue
  DemDebounceBehavior : Constant  Value=[0,0]  OutDataTypeStr=uint8
  Demux{,1..13} (14 alike) : Demux  Outputs=2
  Mux1 : Mux  Inputs=2
  Mux2 : Mux  Inputs=2
  Mux3 : Mux  Inputs=2
  debouncevalue : Outport
  failed : Outport  Port=2
  passed : Outport  Port=3
  wires:
  AEMS_DEM_COUNTER_BASED_DEBOUNCE_THRSHOLD_DYN_CALL2/3(passed) -> Mux3/2
  Mux3/1 -> passed/1
  AEMS_DEM_COUNTER_BASED_DEBOUNCE_THRSHOLD_DYN_CALL1/3(passed) -> Mux3/1
  AEMS_DEM_COUNTER_BASED_DEBOUNCE_THRSHOLD_DYN_CALL2/2(failed) -> Mux2/2
  Mux2/1 -> failed/1
  AEMS_DEM_COUNTER_BASED_DEBOUNCE_THRSHOLD_DYN_CALL1/2(failed) -> Mux2/1
  AEMS_DEM_COUNTER_BASED_DEBOUNCE_THRSHOLD_DYN_CALL2/1(debouncevalue) -> Mux1/2
  Mux1/1 -> debouncevalue/1
  AEMS_DEM_COUNTER_BASED_DEBOUNCE_THRSHOLD_DYN_CALL1/1(debouncevalue) -> Mux1/1
  Demux13/2 -> AEMS_DEM_COUNTER_BASED_DEBOUNCE_THRSHOLD_DYN_CALL2/13(reseteventdebounce)
  Demux13/1 -> AEMS_DEM_COUNTER_BASED_DEBOUNCE_THRSHOLD_DYN_CALL1/13(reseteventdebounce)
  reseteventdebounce/1 -> Demux13/1  "reseteventdebounce"
  Demux12/2 -> AEMS_DEM_COUNTER_BASED_DEBOUNCE_THRSHOLD_DYN_CALL2/12(DemCounterJumpDownValue)
  Demux12/1 -> AEMS_DEM_COUNTER_BASED_DEBOUNCE_THRSHOLD_DYN_CALL1/12(DemCounterJumpDownValue)
  DemCounterJumpDownValue/1 -> Demux12/1  "jumpupvalue_with_prefailed"
  Demux11/2 -> AEMS_DEM_COUNTER_BASED_DEBOUNCE_THRSHOLD_DYN_CALL2/11(DemCounterJumpDown)
  Demux11/1 -> AEMS_DEM_COUNTER_BASED_DEBOUNCE_THRSHOLD_DYN_CALL1/11(DemCounterJumpDown)
  DemCounterJumpDown/1 -> Demux11/1  "jumpdown_activation_with_prepassed"
  Demux10/2 -> AEMS_DEM_COUNTER_BASED_DEBOUNCE_THRSHOLD_DYN_CALL2/10(DemCounterDecrementStepSize)
  Demux10/1 -> AEMS_DEM_COUNTER_BASED_DEBOUNCE_THRSHOLD_DYN_CALL1/10(DemCounterDecrementStepSize)
  DemCounterDecrementStepSize/1 -> Demux10/1  "decrementstepsize_for_prepassed"
  Demux9/2 -> AEMS_DEM_COUNTER_BASED_DEBOUNCE_THRSHOLD_DYN_CALL2/9(passedthreshold)
  Demux9/1 -> AEMS_DEM_COUNTER_BASED_DEBOUNCE_THRSHOLD_DYN_CALL1/9(passedthreshold)
  passedthreshold/1 -> Demux9/1  "passedthreshold"
  Demux8/2 -> AEMS_DEM_COUNTER_BASED_DEBOUNCE_THRSHOLD_DYN_CALL2/8(DemCounterJumpUpValue)
  Demux8/1 -> AEMS_DEM_COUNTER_BASED_DEBOUNCE_THRSHOLD_DYN_CALL1/8(DemCounterJumpUpValue)
  DemCounterJumpUpValue/1 -> Demux8/1  "jumpupvalue_with_prefailed"
  Demux7/2 -> AEMS_DEM_COUNTER_BASED_DEBOUNCE_THRSHOLD_DYN_CALL2/7(DemCounterJumpUp)
  Demux7/1 -> AEMS_DEM_COUNTER_BASED_DEBOUNCE_THRSHOLD_DYN_CALL1/7(DemCounterJumpUp)
  DemCounterJumpUp/1 -> Demux7/1  "jumpup_activation_with_prefailed"
  Demux6/2 -> AEMS_DEM_COUNTER_BASED_DEBOUNCE_THRSHOLD_DYN_CALL2/6(DemCounterIncrementStepSize)
  Demux6/1 -> AEMS_DEM_COUNTER_BASED_DEBOUNCE_THRSHOLD_DYN_CALL1/6(DemCounterIncrementStepSize)
  DemCounterIncrementStepSize/1 -> Demux6/1  "incrementstepsize_for_prefailed"
  Demux5/2 -> AEMS_DEM_COUNTER_BASED_DEBOUNCE_THRSHOLD_DYN_CALL2/5(failedthreshold)
  Demux5/1 -> AEMS_DEM_COUNTER_BASED_DEBOUNCE_THRSHOLD_DYN_CALL1/5(failedthreshold)
  failedthreshold/1 -> Demux5/1  "failedthreshold"
  Demux4/2 -> AEMS_DEM_COUNTER_BASED_DEBOUNCE_THRSHOLD_DYN_CALL2/4(DemDebounceBehavior)
  Demux4/1 -> AEMS_DEM_COUNTER_BASED_DEBOUNCE_THRSHOLD_DYN_CALL1/4(DemDebounceBehavior)
  DemDebounceBehavior/1 -> Demux4/1  "behavior"
  Demux3/2 -> AEMS_DEM_COUNTER_BASED_DEBOUNCE_THRSHOLD_DYN_CALL2/3(prepassed)
  Demux3/1 -> AEMS_DEM_COUNTER_BASED_DEBOUNCE_THRSHOLD_DYN_CALL1/3(prepassed)
  prepassed/1 -> Demux3/1  "prepassed"
  Demux2/2 -> AEMS_DEM_COUNTER_BASED_DEBOUNCE_THRSHOLD_DYN_CALL2/2(prefailed)
  Demux2/1 -> AEMS_DEM_COUNTER_BASED_DEBOUNCE_THRSHOLD_DYN_CALL1/2(prefailed)
  prefailed/1 -> Demux2/1  "prefailed"
  Demux1/2 -> AEMS_DEM_COUNTER_BASED_DEBOUNCE_THRSHOLD_DYN_CALL2/1(conditionfulfilled)
  Demux1/1 -> AEMS_DEM_COUNTER_BASED_DEBOUNCE_THRSHOLD_DYN_CALL1/1(conditionfulfilled)
  conditionfulfilled/1 -> Demux1/1  "conditionfulfilled"
  Demux/2 -> AEMS_DEM_COUNTER_BASED_DEBOUNCE_THRSHOLD_DYN_CALL2/Enable
  Demux/1 -> AEMS_DEM_COUNTER_BASED_DEBOUNCE_THRSHOLD_DYN_CALL1/Enable
  flag_set/1 -> Demux/1

== system AEMS_Standard_Library/SUB/AEMS_DEM_COUNTER_BASED_DEBOUNCE_THRSHOLD_DYN_3D ==
  note: DemDebounceBehavior
  flag_set : Inport
  conditionfulfilled : Inport  Port=2
  prefailed : Inport  Port=3
  prepassed : Inport  Port=4
  failedthreshold : Inport  Port=5
  passedthreshold : Inport  Port=6
  reseteventdebounce : Inport  Port=7
  AEMS_DEM_COUNTER_BASED_DEBOUNCE_THRSHOLD_DYN_CALL1 : Subsystem
  AEMS_DEM_COUNTER_BASED_DEBOUNCE_THRSHOLD_DYN_CALL2 : Subsystem
  AEMS_DEM_COUNTER_BASED_DEBOUNCE_THRSHOLD_DYN_CALL3 : Subsystem
  DemCounterDecrementStepSize : Constant  Value=DemCounterDecrementStepSize
  DemCounterIncrementStepSize : Constant  Value=DemCounterIncrementStepSize
  DemCounterJumpDown : Constant  Value=DemCounterJumpDown
  DemCounterJumpDownValue : Constant  Value=DemCounterJumpDownValue
  DemCounterJumpUp : Constant  Value=DemCounterJumpUp
  DemCounterJumpUpValue : Constant  Value=DemCounterJumpUpValue
  DemDebounceBehavior : Constant  Value=[0,0,0]  OutDataTypeStr=uint8
  Demux{,1..13} (14 alike) : Demux  Outputs=3
  Mux1 : Mux  Inputs=3
  Mux2 : Mux  Inputs=3
  Mux3 : Mux  Inputs=3
  debouncevalue : Outport
  failed : Outport  Port=2
  passed : Outport  Port=3
  wires:
  flag_set/1 -> Demux/1
  Demux/1 -> AEMS_DEM_COUNTER_BASED_DEBOUNCE_THRSHOLD_DYN_CALL1/Enable
  Demux/2 -> AEMS_DEM_COUNTER_BASED_DEBOUNCE_THRSHOLD_DYN_CALL2/Enable
  conditionfulfilled/1 -> Demux1/1  "conditionfulfilled"
  Demux1/1 -> AEMS_DEM_COUNTER_BASED_DEBOUNCE_THRSHOLD_DYN_CALL1/1(conditionfulfilled)
  Demux1/2 -> AEMS_DEM_COUNTER_BASED_DEBOUNCE_THRSHOLD_DYN_CALL2/1(conditionfulfilled)
  prefailed/1 -> Demux2/1  "prefailed"
  Demux2/1 -> AEMS_DEM_COUNTER_BASED_DEBOUNCE_THRSHOLD_DYN_CALL1/2(prefailed)
  Demux2/2 -> AEMS_DEM_COUNTER_BASED_DEBOUNCE_THRSHOLD_DYN_CALL2/2(prefailed)
  prepassed/1 -> Demux3/1  "prepassed"
  Demux3/1 -> AEMS_DEM_COUNTER_BASED_DEBOUNCE_THRSHOLD_DYN_CALL1/3(prepassed)
  Demux3/2 -> AEMS_DEM_COUNTER_BASED_DEBOUNCE_THRSHOLD_DYN_CALL2/3(prepassed)
  DemDebounceBehavior/1 -> Demux4/1  "behavior"
  Demux4/1 -> AEMS_DEM_COUNTER_BASED_DEBOUNCE_THRSHOLD_DYN_CALL1/4(DemDebounceBehavior)
  Demux4/2 -> AEMS_DEM_COUNTER_BASED_DEBOUNCE_THRSHOLD_DYN_CALL2/4(DemDebounceBehavior)
  failedthreshold/1 -> Demux5/1  "failedthreshold"
  Demux5/1 -> AEMS_DEM_COUNTER_BASED_DEBOUNCE_THRSHOLD_DYN_CALL1/5(failedthreshold)
  Demux5/2 -> AEMS_DEM_COUNTER_BASED_DEBOUNCE_THRSHOLD_DYN_CALL2/5(failedthreshold)
  DemCounterIncrementStepSize/1 -> Demux6/1  "incrementstepsize_for_prefailed"
  Demux6/1 -> AEMS_DEM_COUNTER_BASED_DEBOUNCE_THRSHOLD_DYN_CALL1/6(DemCounterIncrementStepSize)
  Demux6/2 -> AEMS_DEM_COUNTER_BASED_DEBOUNCE_THRSHOLD_DYN_CALL2/6(DemCounterIncrementStepSize)
  DemCounterJumpUp/1 -> Demux7/1  "jumpup_activation_with_prefailed"
  Demux7/1 -> AEMS_DEM_COUNTER_BASED_DEBOUNCE_THRSHOLD_DYN_CALL1/7(DemCounterJumpUp)
  Demux7/2 -> AEMS_DEM_COUNTER_BASED_DEBOUNCE_THRSHOLD_DYN_CALL2/7(DemCounterJumpUp)
  DemCounterJumpUpValue/1 -> Demux8/1  "jumpupvalue_with_prefailed"
  Demux8/1 -> AEMS_DEM_COUNTER_BASED_DEBOUNCE_THRSHOLD_DYN_CALL1/8(DemCounterJumpUpValue)
  Demux8/2 -> AEMS_DEM_COUNTER_BASED_DEBOUNCE_THRSHOLD_DYN_CALL2/8(DemCounterJumpUpValue)
  passedthreshold/1 -> Demux9/1  "passedthreshold"
  Demux9/1 -> AEMS_DEM_COUNTER_BASED_DEBOUNCE_THRSHOLD_DYN_CALL1/9(passedthreshold)
  Demux9/2 -> AEMS_DEM_COUNTER_BASED_DEBOUNCE_THRSHOLD_DYN_CALL2/9(passedthreshold)
  DemCounterDecrementStepSize/1 -> Demux10/1  "decrementstepsize_for_prepassed"
  Demux10/1 -> AEMS_DEM_COUNTER_BASED_DEBOUNCE_THRSHOLD_DYN_CALL1/10(DemCounterDecrementStepSize)
  Demux10/2 -> AEMS_DEM_COUNTER_BASED_DEBOUNCE_THRSHOLD_DYN_CALL2/10(DemCounterDecrementStepSize)
  DemCounterJumpDown/1 -> Demux11/1  "jumpdown_activation_with_prepassed"
  Demux11/1 -> AEMS_DEM_COUNTER_BASED_DEBOUNCE_THRSHOLD_DYN_CALL1/11(DemCounterJumpDown)
  Demux11/2 -> AEMS_DEM_COUNTER_BASED_DEBOUNCE_THRSHOLD_DYN_CALL2/11(DemCounterJumpDown)
  DemCounterJumpDownValue/1 -> Demux12/1  "jumpupvalue_with_prefailed"
  Demux12/1 -> AEMS_DEM_COUNTER_BASED_DEBOUNCE_THRSHOLD_DYN_CALL1/12(DemCounterJumpDownValue)
  Demux12/2 -> AEMS_DEM_COUNTER_BASED_DEBOUNCE_THRSHOLD_DYN_CALL2/12(DemCounterJumpDownValue)
  reseteventdebounce/1 -> Demux13/1  "reseteventdebounce"
  Demux13/1 -> AEMS_DEM_COUNTER_BASED_DEBOUNCE_THRSHOLD_DYN_CALL1/13(reseteventdebounce)
  Demux13/2 -> AEMS_DEM_COUNTER_BASED_DEBOUNCE_THRSHOLD_DYN_CALL2/13(reseteventdebounce)
  AEMS_DEM_COUNTER_BASED_DEBOUNCE_THRSHOLD_DYN_CALL1/1(debouncevalue) -> Mux1/1
  Mux1/1 -> debouncevalue/1
  AEMS_DEM_COUNTER_BASED_DEBOUNCE_THRSHOLD_DYN_CALL2/1(debouncevalue) -> Mux1/2
  AEMS_DEM_COUNTER_BASED_DEBOUNCE_THRSHOLD_DYN_CALL1/2(failed) -> Mux2/1
  Mux2/1 -> failed/1
  AEMS_DEM_COUNTER_BASED_DEBOUNCE_THRSHOLD_DYN_CALL2/2(failed) -> Mux2/2
  AEMS_DEM_COUNTER_BASED_DEBOUNCE_THRSHOLD_DYN_CALL1/3(passed) -> Mux3/1
  Mux3/1 -> passed/1
  AEMS_DEM_COUNTER_BASED_DEBOUNCE_THRSHOLD_DYN_CALL2/3(passed) -> Mux3/2
  Demux/3 -> AEMS_DEM_COUNTER_BASED_DEBOUNCE_THRSHOLD_DYN_CALL3/Enable
  Demux1/3 -> AEMS_DEM_COUNTER_BASED_DEBOUNCE_THRSHOLD_DYN_CALL3/1(conditionfulfilled)
  Demux2/3 -> AEMS_DEM_COUNTER_BASED_DEBOUNCE_THRSHOLD_DYN_CALL3/2(prefailed)
  Demux3/3 -> AEMS_DEM_COUNTER_BASED_DEBOUNCE_THRSHOLD_DYN_CALL3/3(prepassed)
  Demux4/3 -> AEMS_DEM_COUNTER_BASED_DEBOUNCE_THRSHOLD_DYN_CALL3/4(DemDebounceBehavior)
  Demux5/3 -> AEMS_DEM_COUNTER_BASED_DEBOUNCE_THRSHOLD_DYN_CALL3/5(failedthreshold)
  Demux6/3 -> AEMS_DEM_COUNTER_BASED_DEBOUNCE_THRSHOLD_DYN_CALL3/6(DemCounterIncrementStepSize)
  Demux7/3 -> AEMS_DEM_COUNTER_BASED_DEBOUNCE_THRSHOLD_DYN_CALL3/7(DemCounterJumpUp)
  Demux8/3 -> AEMS_DEM_COUNTER_BASED_DEBOUNCE_THRSHOLD_DYN_CALL3/8(DemCounterJumpUpValue)
  Demux9/3 -> AEMS_DEM_COUNTER_BASED_DEBOUNCE_THRSHOLD_DYN_CALL3/9(passedthreshold)
  Demux10/3 -> AEMS_DEM_COUNTER_BASED_DEBOUNCE_THRSHOLD_DYN_CALL3/10(DemCounterDecrementStepSize)
  Demux11/3 -> AEMS_DEM_COUNTER_BASED_DEBOUNCE_THRSHOLD_DYN_CALL3/11(DemCounterJumpDown)
  Demux12/3 -> AEMS_DEM_COUNTER_BASED_DEBOUNCE_THRSHOLD_DYN_CALL3/12(DemCounterJumpDownValue)
  Demux13/3 -> AEMS_DEM_COUNTER_BASED_DEBOUNCE_THRSHOLD_DYN_CALL3/13(reseteventdebounce)
  AEMS_DEM_COUNTER_BASED_DEBOUNCE_THRSHOLD_DYN_CALL3/1(debouncevalue) -> Mux1/3
  AEMS_DEM_COUNTER_BASED_DEBOUNCE_THRSHOLD_DYN_CALL3/2(failed) -> Mux2/3
  AEMS_DEM_COUNTER_BASED_DEBOUNCE_THRSHOLD_DYN_CALL3/3(passed) -> Mux3/3

== system AEMS_Standard_Library/SUB/AEMS_DEM_COUNTER_BASED_DEBOUNCE_THRSHOLD_DYN_4D ==
  note: DemDebounceBehavior
  flag_set : Inport
  conditionfulfilled : Inport  Port=2
  prefailed : Inport  Port=3
  prepassed : Inport  Port=4
  failedthreshold : Inport  Port=5
  passedthreshold : Inport  Port=6
  reseteventdebounce : Inport  Port=7
  AEMS_DEM_COUNTER_BASED_DEBOUNCE_THRSHOLD_DYN_CALL1 : Subsystem
  AEMS_DEM_COUNTER_BASED_DEBOUNCE_THRSHOLD_DYN_CALL2 : Subsystem
  AEMS_DEM_COUNTER_BASED_DEBOUNCE_THRSHOLD_DYN_CALL3 : Subsystem
  AEMS_DEM_COUNTER_BASED_DEBOUNCE_THRSHOLD_DYN_CALL4 : Subsystem
  DemCounterDecrementStepSize : Constant  Value=DemCounterDecrementStepSize
  DemCounterIncrementStepSize : Constant  Value=DemCounterIncrementStepSize
  DemCounterJumpDown : Constant  Value=DemCounterJumpDown
  DemCounterJumpDownValue : Constant  Value=DemCounterJumpDownValue
  DemCounterJumpUp : Constant  Value=DemCounterJumpUp
  DemCounterJumpUpValue : Constant  Value=DemCounterJumpUpValue
  DemDebounceBehavior : Constant  Value=[0,0,0,0]  OutDataTypeStr=uint8
  Demux{,1..13} (14 alike) : Demux
  Mux1 : Mux
  Mux2 : Mux
  Mux3 : Mux
  debouncevalue : Outport
  failed : Outport  Port=2
  passed : Outport  Port=3
  wires:
  flag_set/1 -> Demux/1
  Demux/1 -> AEMS_DEM_COUNTER_BASED_DEBOUNCE_THRSHOLD_DYN_CALL1/Enable
  Demux/2 -> AEMS_DEM_COUNTER_BASED_DEBOUNCE_THRSHOLD_DYN_CALL2/Enable
  conditionfulfilled/1 -> Demux1/1  "conditionfulfilled"
  Demux1/1 -> AEMS_DEM_COUNTER_BASED_DEBOUNCE_THRSHOLD_DYN_CALL1/1(conditionfulfilled)
  Demux1/2 -> AEMS_DEM_COUNTER_BASED_DEBOUNCE_THRSHOLD_DYN_CALL2/1(conditionfulfilled)
  prefailed/1 -> Demux2/1  "prefailed"
  Demux2/1 -> AEMS_DEM_COUNTER_BASED_DEBOUNCE_THRSHOLD_DYN_CALL1/2(prefailed)
  Demux2/2 -> AEMS_DEM_COUNTER_BASED_DEBOUNCE_THRSHOLD_DYN_CALL2/2(prefailed)
  prepassed/1 -> Demux3/1  "prepassed"
  Demux3/1 -> AEMS_DEM_COUNTER_BASED_DEBOUNCE_THRSHOLD_DYN_CALL1/3(prepassed)
  Demux3/2 -> AEMS_DEM_COUNTER_BASED_DEBOUNCE_THRSHOLD_DYN_CALL2/3(prepassed)
  DemDebounceBehavior/1 -> Demux4/1  "behavior"
  Demux4/1 -> AEMS_DEM_COUNTER_BASED_DEBOUNCE_THRSHOLD_DYN_CALL1/4(DemDebounceBehavior)
  Demux4/2 -> AEMS_DEM_COUNTER_BASED_DEBOUNCE_THRSHOLD_DYN_CALL2/4(DemDebounceBehavior)
  failedthreshold/1 -> Demux5/1  "failedthreshold"
  Demux5/1 -> AEMS_DEM_COUNTER_BASED_DEBOUNCE_THRSHOLD_DYN_CALL1/5(failedthreshold)
  Demux5/2 -> AEMS_DEM_COUNTER_BASED_DEBOUNCE_THRSHOLD_DYN_CALL2/5(failedthreshold)
  DemCounterIncrementStepSize/1 -> Demux6/1  "incrementstepsize_for_prefailed"
  Demux6/1 -> AEMS_DEM_COUNTER_BASED_DEBOUNCE_THRSHOLD_DYN_CALL1/6(DemCounterIncrementStepSize)
  Demux6/2 -> AEMS_DEM_COUNTER_BASED_DEBOUNCE_THRSHOLD_DYN_CALL2/6(DemCounterIncrementStepSize)
  DemCounterJumpUp/1 -> Demux7/1  "jumpup_activation_with_prefailed"
  Demux7/1 -> AEMS_DEM_COUNTER_BASED_DEBOUNCE_THRSHOLD_DYN_CALL1/7(DemCounterJumpUp)
  Demux7/2 -> AEMS_DEM_COUNTER_BASED_DEBOUNCE_THRSHOLD_DYN_CALL2/7(DemCounterJumpUp)
  DemCounterJumpUpValue/1 -> Demux8/1  "jumpupvalue_with_prefailed"
  Demux8/1 -> AEMS_DEM_COUNTER_BASED_DEBOUNCE_THRSHOLD_DYN_CALL1/8(DemCounterJumpUpValue)
  Demux8/2 -> AEMS_DEM_COUNTER_BASED_DEBOUNCE_THRSHOLD_DYN_CALL2/8(DemCounterJumpUpValue)
  passedthreshold/1 -> Demux9/1  "passedthreshold"
  Demux9/1 -> AEMS_DEM_COUNTER_BASED_DEBOUNCE_THRSHOLD_DYN_CALL1/9(passedthreshold)
  Demux9/2 -> AEMS_DEM_COUNTER_BASED_DEBOUNCE_THRSHOLD_DYN_CALL2/9(passedthreshold)
  DemCounterDecrementStepSize/1 -> Demux10/1  "decrementstepsize_for_prepassed"
  Demux10/1 -> AEMS_DEM_COUNTER_BASED_DEBOUNCE_THRSHOLD_DYN_CALL1/10(DemCounterDecrementStepSize)
  Demux10/2 -> AEMS_DEM_COUNTER_BASED_DEBOUNCE_THRSHOLD_DYN_CALL2/10(DemCounterDecrementStepSize)
  DemCounterJumpDown/1 -> Demux11/1  "jumpdown_activation_with_prepassed"
  Demux11/1 -> AEMS_DEM_COUNTER_BASED_DEBOUNCE_THRSHOLD_DYN_CALL1/11(DemCounterJumpDown)
  Demux11/2 -> AEMS_DEM_COUNTER_BASED_DEBOUNCE_THRSHOLD_DYN_CALL2/11(DemCounterJumpDown)
  DemCounterJumpDownValue/1 -> Demux12/1  "jumpupvalue_with_prefailed"
  Demux12/1 -> AEMS_DEM_COUNTER_BASED_DEBOUNCE_THRSHOLD_DYN_CALL1/12(DemCounterJumpDownValue)
  Demux12/2 -> AEMS_DEM_COUNTER_BASED_DEBOUNCE_THRSHOLD_DYN_CALL2/12(DemCounterJumpDownValue)
  reseteventdebounce/1 -> Demux13/1  "reseteventdebounce"
  Demux13/1 -> AEMS_DEM_COUNTER_BASED_DEBOUNCE_THRSHOLD_DYN_CALL1/13(reseteventdebounce)
  Demux13/2 -> AEMS_DEM_COUNTER_BASED_DEBOUNCE_THRSHOLD_DYN_CALL2/13(reseteventdebounce)
  AEMS_DEM_COUNTER_BASED_DEBOUNCE_THRSHOLD_DYN_CALL1/1(debouncevalue) -> Mux1/1
  Mux1/1 -> debouncevalue/1
  AEMS_DEM_COUNTER_BASED_DEBOUNCE_THRSHOLD_DYN_CALL2/1(debouncevalue) -> Mux1/2
  AEMS_DEM_COUNTER_BASED_DEBOUNCE_THRSHOLD_DYN_CALL1/2(failed) -> Mux2/1
  Mux2/1 -> failed/1
  AEMS_DEM_COUNTER_BASED_DEBOUNCE_THRSHOLD_DYN_CALL2/2(failed) -> Mux2/2
  AEMS_DEM_COUNTER_BASED_DEBOUNCE_THRSHOLD_DYN_CALL1/3(passed) -> Mux3/1
  Mux3/1 -> passed/1
  AEMS_DEM_COUNTER_BASED_DEBOUNCE_THRSHOLD_DYN_CALL2/3(passed) -> Mux3/2
  Demux/3 -> AEMS_DEM_COUNTER_BASED_DEBOUNCE_THRSHOLD_DYN_CALL3/Enable
  Demux1/3 -> AEMS_DEM_COUNTER_BASED_DEBOUNCE_THRSHOLD_DYN_CALL3/1(conditionfulfilled)
  Demux2/3 -> AEMS_DEM_COUNTER_BASED_DEBOUNCE_THRSHOLD_DYN_CALL3/2(prefailed)
  Demux3/3 -> AEMS_DEM_COUNTER_BASED_DEBOUNCE_THRSHOLD_DYN_CALL3/3(prepassed)
  Demux4/3 -> AEMS_DEM_COUNTER_BASED_DEBOUNCE_THRSHOLD_DYN_CALL3/4(DemDebounceBehavior)
  Demux5/3 -> AEMS_DEM_COUNTER_BASED_DEBOUNCE_THRSHOLD_DYN_CALL3/5(failedthreshold)
  Demux6/3 -> AEMS_DEM_COUNTER_BASED_DEBOUNCE_THRSHOLD_DYN_CALL3/6(DemCounterIncrementStepSize)
  Demux7/3 -> AEMS_DEM_COUNTER_BASED_DEBOUNCE_THRSHOLD_DYN_CALL3/7(DemCounterJumpUp)
  Demux8/3 -> AEMS_DEM_COUNTER_BASED_DEBOUNCE_THRSHOLD_DYN_CALL3/8(DemCounterJumpUpValue)
  Demux9/3 -> AEMS_DEM_COUNTER_BASED_DEBOUNCE_THRSHOLD_DYN_CALL3/9(passedthreshold)
  Demux10/3 -> AEMS_DEM_COUNTER_BASED_DEBOUNCE_THRSHOLD_DYN_CALL3/10(DemCounterDecrementStepSize)
  Demux11/3 -> AEMS_DEM_COUNTER_BASED_DEBOUNCE_THRSHOLD_DYN_CALL3/11(DemCounterJumpDown)
  Demux12/3 -> AEMS_DEM_COUNTER_BASED_DEBOUNCE_THRSHOLD_DYN_CALL3/12(DemCounterJumpDownValue)
  Demux13/3 -> AEMS_DEM_COUNTER_BASED_DEBOUNCE_THRSHOLD_DYN_CALL3/13(reseteventdebounce)
  AEMS_DEM_COUNTER_BASED_DEBOUNCE_THRSHOLD_DYN_CALL3/1(debouncevalue) -> Mux1/3
  AEMS_DEM_COUNTER_BASED_DEBOUNCE_THRSHOLD_DYN_CALL3/2(failed) -> Mux2/3
  AEMS_DEM_COUNTER_BASED_DEBOUNCE_THRSHOLD_DYN_CALL3/3(passed) -> Mux3/3
  Demux/4 -> AEMS_DEM_COUNTER_BASED_DEBOUNCE_THRSHOLD_DYN_CALL4/Enable
  Demux1/4 -> AEMS_DEM_COUNTER_BASED_DEBOUNCE_THRSHOLD_DYN_CALL4/1(conditionfulfilled)
  Demux2/4 -> AEMS_DEM_COUNTER_BASED_DEBOUNCE_THRSHOLD_DYN_CALL4/2(prefailed)
  Demux3/4 -> AEMS_DEM_COUNTER_BASED_DEBOUNCE_THRSHOLD_DYN_CALL4/3(prepassed)
  Demux4/4 -> AEMS_DEM_COUNTER_BASED_DEBOUNCE_THRSHOLD_DYN_CALL4/4(DemDebounceBehavior)
  Demux5/4 -> AEMS_DEM_COUNTER_BASED_DEBOUNCE_THRSHOLD_DYN_CALL4/5(failedthreshold)
  Demux6/4 -> AEMS_DEM_COUNTER_BASED_DEBOUNCE_THRSHOLD_DYN_CALL4/6(DemCounterIncrementStepSize)
  Demux7/4 -> AEMS_DEM_COUNTER_BASED_DEBOUNCE_THRSHOLD_DYN_CALL4/7(DemCounterJumpUp)
  Demux8/4 -> AEMS_DEM_COUNTER_BASED_DEBOUNCE_THRSHOLD_DYN_CALL4/8(DemCounterJumpUpValue)
  Demux9/4 -> AEMS_DEM_COUNTER_BASED_DEBOUNCE_THRSHOLD_DYN_CALL4/9(passedthreshold)
  Demux10/4 -> AEMS_DEM_COUNTER_BASED_DEBOUNCE_THRSHOLD_DYN_CALL4/10(DemCounterDecrementStepSize)
  Demux11/4 -> AEMS_DEM_COUNTER_BASED_DEBOUNCE_THRSHOLD_DYN_CALL4/11(DemCounterJumpDown)
  Demux12/4 -> AEMS_DEM_COUNTER_BASED_DEBOUNCE_THRSHOLD_DYN_CALL4/12(DemCounterJumpDownValue)
  Demux13/4 -> AEMS_DEM_COUNTER_BASED_DEBOUNCE_THRSHOLD_DYN_CALL4/13(reseteventdebounce)
  AEMS_DEM_COUNTER_BASED_DEBOUNCE_THRSHOLD_DYN_CALL4/1(debouncevalue) -> Mux1/4
  AEMS_DEM_COUNTER_BASED_DEBOUNCE_THRSHOLD_DYN_CALL4/2(failed) -> Mux2/4
  AEMS_DEM_COUNTER_BASED_DEBOUNCE_THRSHOLD_DYN_CALL4/3(passed) -> Mux3/4
